simulink model "sf_aircraft"  (Simulink 7.6)
settings: Solver=ode4  StartTime=0.0  StopTime=inf  RelTol=1e-3
PreLoadFcn:
  | noise_factor=1;
  | load sf_aircraft_buses;
undefined symbols (not defined in the file or in its folder): sf_aircraft_ModeType, sigbuilder_block
libraries: simulink x21, sf_aircraft_screen_library x7, simulink_need_slupdate x2
(part 2 of 2)

== system sf_aircraft/Signal conditioning and failures /Actuator Positions/Event Logging/Log LI Actuator  Position Sensors ==
  In1 : Inport
  Enable : EnablePort  PropagateVarSize=During execution
  To Workspace : ToWorkspace  VariableName=LI_log  SampleTime=-1  SaveFormat=Structure With Time
  wires:
  In1/1 -> To Workspace/1  "LI_log"

== system sf_aircraft/Signal conditioning and failures /Actuator Positions/Event Logging/Log LO Actuator  Position Sensors ==
  In1 : Inport
  Enable : EnablePort  PropagateVarSize=During execution
  To Workspace : ToWorkspace  VariableName=LO_log  SampleTime=-1  SaveFormat=Structure With Time
  wires:
  In1/1 -> To Workspace/1  "LO_log"

== system sf_aircraft/Signal conditioning and failures /Actuator Positions/Event Logging/Log RI Actuator  Position Sensors ==
  In1 : Inport
  Enable : EnablePort  PropagateVarSize=During execution
  To Workspace : ToWorkspace  VariableName=RI_log  SampleTime=-1  SaveFormat=Structure With Time
  wires:
  In1/1 -> To Workspace/1  "RO_log"

== system sf_aircraft/Signal conditioning and failures /Actuator Positions/Event Logging/Log RO Actuator  Position Sensors ==
  In1 : Inport
  Enable : EnablePort  PropagateVarSize=During execution
  To Workspace : ToWorkspace  VariableName=RO_log  SampleTime=-1  SaveFormat=Structure With Time
  wires:
  In1/1 -> To Workspace/1  "RI_log"

== system sf_aircraft/Signal conditioning and failures /Hydraulic Pressures/Event Logging/Log Hydraulic System 1 Sensors ==
  In1 : Inport
  Enable : EnablePort  PropagateVarSize=During execution
  To Workspace : ToWorkspace  VariableName=H1_log  SampleTime=-1  SaveFormat=Structure With Time
  wires:
  In1/1 -> To Workspace/1

== system sf_aircraft/Signal conditioning and failures /Hydraulic Pressures/Event Logging/Log Hydraulic System 2 Sensors ==
  In1 : Inport
  Enable : EnablePort  PropagateVarSize=During execution
  To Workspace : ToWorkspace  VariableName=H2_log  SampleTime=-1  SaveFormat=Structure With Time
  wires:
  In1/1 -> To Workspace/1  "H2_log"

== system sf_aircraft/Signal conditioning and failures /Hydraulic Pressures/Event Logging/Log Hydraulic System 3 Sensors ==
  In1 : Inport
  Enable : EnablePort  PropagateVarSize=During execution
  To Workspace : ToWorkspace  VariableName=H3_log  SampleTime=-1  SaveFormat=Structure With Time
  wires:
  In1/1 -> To Workspace/1  "H3_log"

== system sf_aircraft/Signal conditioning and failures /Hydraulic Pressures/Measured  Hydraulic system 1 pressures/Hydraulic pressure ==
  H1_fail : Constant  Value=0  OutDataTypeStr=boolean
  Outlier/failure : Subsystem  Tag=STV Subsys  LoadFcn=sigbuilder_block('load');  StartFcn=sigbuilder_block('start');  StopFcn=sigbuilder_block('stop');  ClipboardFcn=sigbuilder_block('clipboard');  mask(Sigbuilder block){}
      mask help: Sigbuilder GUI
      mask init:
      | if ~strcmp(get_param(bdroot,'SimulationStatus'),'stopped') tuvar = sigbuilder_block('maskInit'); end
      settings: CopyFcn=sigbuilder_block('copy');  DeleteFcn=sigbuilder_block('delete');  ModelCloseFcn=sigbuilder_block('modelClose');  PreSaveFcn=sigbuilder_block('preSave');  NameChangeFcn=sigbuilder_block('namechange');  OpenFcn=sigbuilder_block('open',[81 97.5 519.75 399.75 ]);  CloseFcn=sigbuilder_block('close');
      mask Display: plot(0,0,100,100,[10,10,40,40,10],[80,20,20,80,80],[40,10],[50,50], [40,27,10],[65,72,56],[40,25,25,10],[28,28,43,43]);
  Pump Pressure : Constant  Value=1000
  Switch : Switch  Criteria=u2 ~= 0  SaturateOnIntegerOverflow=on
  Out1 : Outport
  wires:
  Pump Pressure/1 -> Switch/3
  Switch/1 -> Out1/1
  Outlier/failure/1(Signal 1) -> Switch/1
  H1_fail/1 -> Switch/2

== system sf_aircraft/Signal conditioning and failures /Hydraulic Pressures/Measured  Hydraulic system 1 pressures/pressure reading1 ==
  pressure : Inport
  Band-Limited White Noise : simulink/Sources/Band-Limited White Noise  SystemSampleTime=-1  Cov=[0.1]*noise_factor  Ts=0.01  seed=[25341]
  Sum : Sum  Inputs=|++  SaturateOnIntegerOverflow=on
  Out1 : Outport
  wires:
  Sum/1 -> Out1/1
  pressure/1 -> Sum/1
  Band-Limited White Noise/1 -> Sum/2

== system sf_aircraft/Signal conditioning and failures /Hydraulic Pressures/Measured  Hydraulic system 1 pressures/pressure reading2 ==
  pressure : Inport
  Band-Limited White Noise : simulink/Sources/Band-Limited White Noise  SystemSampleTime=-1  Cov=[0.1]*noise_factor  Ts=0.01  seed=[21311]
  Sum1 : Sum  Inputs=|++  SaturateOnIntegerOverflow=on
  Out1 : Outport
  wires:
  Band-Limited White Noise/1 -> Sum1/2
  pressure/1 -> Sum1/1
  Sum1/1 -> Out1/1

== system sf_aircraft/Signal conditioning and failures /Hydraulic Pressures/Measured  Hydraulic system 1 pressures/pressure reading3 ==
  pressure : Inport
  Band-Limited White Noise : simulink/Sources/Band-Limited White Noise  SystemSampleTime=-1  Cov=[0.1]*noise_factor  Ts=0.01  seed=[341]
  Sum1 : Sum  Inputs=|++  SaturateOnIntegerOverflow=on
  Out1 : Outport
  wires:
  Sum1/1 -> Out1/1
  pressure/1 -> Sum1/1
  Band-Limited White Noise/1 -> Sum1/2

== system sf_aircraft/Signal conditioning and failures /Hydraulic Pressures/Measured  Hydraulic system 2 pressures/Hydraulic pressure ==
  H2_fail : Constant  Value=0  OutDataTypeStr=boolean
  Outlier/failure : Subsystem  Tag=STV Subsys  LoadFcn=sigbuilder_block('load');  StartFcn=sigbuilder_block('start');  StopFcn=sigbuilder_block('stop');  ClipboardFcn=sigbuilder_block('clipboard');  mask(Sigbuilder block){}
      mask help: Sigbuilder GUI
      mask init:
      | if ~strcmp(get_param(bdroot,'SimulationStatus'),'stopped') tuvar = sigbuilder_block('maskInit'); end
      settings: CopyFcn=sigbuilder_block('copy');  DeleteFcn=sigbuilder_block('delete');  ModelCloseFcn=sigbuilder_block('modelClose');  PreSaveFcn=sigbuilder_block('preSave');  NameChangeFcn=sigbuilder_block('namechange');  OpenFcn=sigbuilder_block('open',[81 97.5 519.75 399.75 ]);  CloseFcn=sigbuilder_block('close');
      mask Display: plot(0,0,100,100,[10,10,40,40,10],[80,20,20,80,80],[40,10],[50,50], [40,27,10],[65,72,56],[40,25,25,10],[28,28,43,43]);
  Pump Pressure : Constant  Value=1000
  Switch : Switch  Criteria=u2 ~= 0  SaturateOnIntegerOverflow=on
  Out1 : Outport
  wires:
  Pump Pressure/1 -> Switch/3
  Switch/1 -> Out1/1
  Outlier/failure/1(Signal 1) -> Switch/1
  H2_fail/1 -> Switch/2

== system sf_aircraft/Signal conditioning and failures /Hydraulic Pressures/Measured  Hydraulic system 2 pressures/pressure reading1 ==
  pressure : Inport
  Band-Limited White Noise : simulink/Sources/Band-Limited White Noise  SystemSampleTime=-1  Cov=[0.1]*noise_factor  Ts=0.01  seed=[25341]
  Sum : Sum  Inputs=|++  SaturateOnIntegerOverflow=on
  Out1 : Outport
  wires:
  Band-Limited White Noise/1 -> Sum/2
  pressure/1 -> Sum/1
  Sum/1 -> Out1/1

== system sf_aircraft/Signal conditioning and failures /Hydraulic Pressures/Measured  Hydraulic system 2 pressures/pressure reading2 ==
  pressure : Inport
  Band-Limited White Noise : simulink/Sources/Band-Limited White Noise  SystemSampleTime=-1  Cov=[0.1]*noise_factor  Ts=0.01  seed=[21311]
  Sum1 : Sum  Inputs=|++  SaturateOnIntegerOverflow=on
  Out1 : Outport
  wires:
  Sum1/1 -> Out1/1
  pressure/1 -> Sum1/1
  Band-Limited White Noise/1 -> Sum1/2

== system sf_aircraft/Signal conditioning and failures /Hydraulic Pressures/Measured  Hydraulic system 2 pressures/pressure reading3 ==
  pressure : Inport
  Band-Limited White Noise : simulink/Sources/Band-Limited White Noise  SystemSampleTime=-1  Cov=[0.1]*noise_factor  Ts=0.01  seed=[341]
  Sum1 : Sum  Inputs=|++  SaturateOnIntegerOverflow=on
  Out1 : Outport
  wires:
  Band-Limited White Noise/1 -> Sum1/2
  pressure/1 -> Sum1/1
  Sum1/1 -> Out1/1

== system sf_aircraft/Signal conditioning and failures /Hydraulic Pressures/Measured  Hydraulic system 3 pressures/Hydraulic pressure ==
  H3_fail : Constant  Value=0  OutDataTypeStr=boolean
  Outlier/failure : Subsystem  Tag=STV Subsys  LoadFcn=sigbuilder_block('load');  StartFcn=sigbuilder_block('start');  StopFcn=sigbuilder_block('stop');  ClipboardFcn=sigbuilder_block('clipboard');  mask(Sigbuilder block){}
      mask help: Sigbuilder GUI
      mask init:
      | if ~strcmp(get_param(bdroot,'SimulationStatus'),'stopped') tuvar = sigbuilder_block('maskInit'); end
      settings: CopyFcn=sigbuilder_block('copy');  DeleteFcn=sigbuilder_block('delete');  ModelCloseFcn=sigbuilder_block('modelClose');  PreSaveFcn=sigbuilder_block('preSave');  NameChangeFcn=sigbuilder_block('namechange');  OpenFcn=sigbuilder_block('open',[81 97.5 519.75 399.75 ]);  CloseFcn=sigbuilder_block('close');
      mask Display: plot(0,0,100,100,[10,10,40,40,10],[80,20,20,80,80],[40,10],[50,50], [40,27,10],[65,72,56],[40,25,25,10],[28,28,43,43]);
  Pump Pressure : Constant  Value=1000
  Switch : Switch  Criteria=u2 ~= 0  SaturateOnIntegerOverflow=on
  Out1 : Outport
  wires:
  Pump Pressure/1 -> Switch/3
  Switch/1 -> Out1/1
  Outlier/failure/1(Signal 1) -> Switch/1
  H3_fail/1 -> Switch/2

== system sf_aircraft/Signal conditioning and failures /Hydraulic Pressures/Measured  Hydraulic system 3 pressures/pressure reading1 ==
  pressure : Inport
  Band-Limited White Noise : simulink/Sources/Band-Limited White Noise  SystemSampleTime=-1  Cov=[0.1]*noise_factor  Ts=0.01  seed=[2341]
  Sum : Sum  Inputs=|++  SaturateOnIntegerOverflow=on
  Out1 : Outport
  wires:
  Sum/1 -> Out1/1
  pressure/1 -> Sum/1
  Band-Limited White Noise/1 -> Sum/2

== system sf_aircraft/Signal conditioning and failures /Hydraulic Pressures/Measured  Hydraulic system 3 pressures/pressure reading2 ==
  pressure : Inport
  Band-Limited White Noise : simulink/Sources/Band-Limited White Noise  SystemSampleTime=-1  Cov=[0.1]*noise_factor  Ts=0.01  seed=[1311]
  Sum1 : Sum  Inputs=|++  SaturateOnIntegerOverflow=on
  Out1 : Outport
  wires:
  Band-Limited White Noise/1 -> Sum1/2
  pressure/1 -> Sum1/1
  Sum1/1 -> Out1/1

== system sf_aircraft/Signal conditioning and failures /Hydraulic Pressures/Measured  Hydraulic system 3 pressures/pressure reading3 ==
  pressure : Inport
  Band-Limited White Noise : simulink/Sources/Band-Limited White Noise  SystemSampleTime=-1  Cov=[0.1]*noise_factor  Ts=0.01  seed=[1341]
  Sum1 : Sum  Inputs=|++  SaturateOnIntegerOverflow=on
  Out1 : Outport
  wires:
  Sum1/1 -> Out1/1
  pressure/1 -> Sum1/1
  Band-Limited White Noise/1 -> Sum1/2

== system sf_aircraft/Signal conditioning and failures /Hydraulic Pressures/Measured  Hydraulic system 1 pressures/Hydraulic pressure/Outlier/failure ==
  Demux : Demux  Tag=STV Demux  Outputs=1
  FromWs : FromWorkspace  Tag=STV FromWs  VariableName=tuvar  SampleTime=0  SigBuilderData=DataTag8  VnvData=DataTag9
      SigBuilderData=|
      | dataSet.timeRange = [0 30]
      | dataSet.name = 'Group 1'
      | sbobj.Groups.Name = 'Group 1'
      | sbobj.Groups.Signals.Name = 'Signal 1'
      | sbobj.Groups.Signals.XData = [0 30]
      | sbobj.Groups.Signals.YData = [100 100]
      | sbobj.Groups.TimeRange = [0 30]
  Signal 1 : Outport  Tag=STV Outport
  wires:
  FromWs/1 -> Demux/1
  Demux/1 -> Signal 1/1

== system sf_aircraft/Signal conditioning and failures /Hydraulic Pressures/Measured  Hydraulic system 2 pressures/Hydraulic pressure/Outlier/failure ==
  Demux : Demux  Tag=STV Demux  Outputs=1
  FromWs : FromWorkspace  Tag=STV FromWs  VariableName=tuvar  SampleTime=0  SigBuilderData=DataTag10  VnvData=DataTag11
      SigBuilderData=|
      | dataSet.timeRange = [0 30]
      | dataSet.name = 'Group 1'
      | sbobj.Groups.Name = 'Group 1'
      | sbobj.Groups.Signals.Name = 'Signal 1'
      | sbobj.Groups.Signals.XData = [0 30]
      | sbobj.Groups.Signals.YData = [100 100]
      | sbobj.Groups.TimeRange = [0 30]
  Signal 1 : Outport  Tag=STV Outport
  wires:
  FromWs/1 -> Demux/1
  Demux/1 -> Signal 1/1

== system sf_aircraft/Signal conditioning and failures /Hydraulic Pressures/Measured  Hydraulic system 3 pressures/Hydraulic pressure/Outlier/failure ==
  Demux : Demux  Tag=STV Demux  Outputs=1
  FromWs : FromWorkspace  Tag=STV FromWs  VariableName=tuvar  SampleTime=0  SigBuilderData=DataTag12  VnvData=DataTag13
      SigBuilderData=|
      | dataSet.timeRange = [0 30]
      | dataSet.name = 'Group 1'
      | sbobj.Groups.Name = 'Group 1'
      | sbobj.Groups.Signals.Name = 'Signal 1'
      | sbobj.Groups.Signals.XData = [0 30]
      | sbobj.Groups.Signals.YData = [100 100]
      | sbobj.Groups.TimeRange = [0 30]
  Signal 1 : Outport  Tag=STV Outport
  wires:
  FromWs/1 -> Demux/1
  Demux/1 -> Signal 1/1

== stateflow chart Mode Logic ==
  settings: sampleTime=0.5
  state R_switch [function]
    (default) -> (junction 78)
    (junction 78) -> (junction 79) : {
        | /* Hydraulic system 3 Low pressure (Right Outer line) */
        | aVarTruthTableCondition_1 = (u.low_press[2]);
        | }
    (junction 79) -> (junction 80) : {
        | /* Right Outer actuator position failed */
        | aVarTruthTableCondition_2 = (u.R_pos_fail[0]);
        | }
    (junction 80) -> (junction 81) : {
        | /* Hydraulic system 2 Low pressure (Inner line) */
        | aVarTruthTableCondition_3 = (u.low_press[1]);
        | }
    (junction 81) -> (junction 82) : {
        | /* Right Inner actuator position failed */
        | aVarTruthTableCondition_4 = (u.R_pos_fail[1]);
        | }
    (junction 82) -> (junction 83) [order 1] : [aVarTruthTableCondition_1 && !aVarTruthTableCondition_3 && !aVarTruthTableCondition_4]
    (junction 83) -> (junction 84) : {
        | /* Hydraulic System 3 Failure. Turn off Right Outer Actuator */
        | send(go_off,Actuators.RO);
        | }
    (junction 82) -> (junction 85) [order 2]
    (junction 85) -> (junction 86) [order 1] : [aVarTruthTableCondition_1]
    (junction 86) -> (junction 87) : {
        | /* Mulitple Failure. Isolate Right Outer AND Right Inner Actuators */
        | send(go_isolated,Actuators.RO);
        | send(go_isolated,Actuators.RI);
        | }
    (junction 85) -> (junction 88) [order 2]
    (junction 88) -> (junction 89) [order 1] : [!aVarTruthTableCondition_1 && aVarTruthTableCondition_2 && !aVarTruthTableCondition_3 && !aVarTruthTableCondition_4]
    (junction 89) -> (junction 90) : {
        | /* Right Outer Actuator Failure. Isolate Right Outer Actuator */
        | send(go_isolated,Actuators.RO);
        | }
    (junction 88) -> (junction 91) [order 2]
    (junction 91) -> (junction 92) [order 1] : [!aVarTruthTableCondition_1 && aVarTruthTableCondition_2]
    (junction 92) -> (junction 93) : {
        | /* Mulitple Failure. Isolate Right Outer AND Right Inner Actuators */
        | send(go_isolated,Actuators.RO);
        | send(go_isolated,Actuators.RI);
        | }
    (junction 91) -> (junction 94) [order 2]
    (junction 94) -> (junction 95) [order 1] : [aVarTruthTableCondition_3]
    (junction 95) -> (junction 96) : {
        | /* Hydraulic System 2 Failure. Turn off Right Inner Actuator */
        | send(go_off,Actuators.RI);
        | }
    (junction 94) -> (junction 97) [order 2]
    (junction 97) -> (junction 98) [order 1] : [aVarTruthTableCondition_4]
    (junction 98) -> (junction 99) : {
        | /* Right Inner Actuator Failure. Isolate Right Inner Actuator */
        | send(go_isolated,Actuators.RI);
        | }
    (junction 97) -> (junction 100) [order 2]
    (junction 100) -> (junction 101) : /* Default */
    (junction 101) -> (junction 102) : {
        | /* 'Default':Default - All ok, do nothing. */
        |
        | }
  state Actuators
    en:L_switch();R_switch();
    du:L_switch();R_switch();
    state LO [parallel]
      settings: executionOrder=1
      state L1
        state passive
          y.LO_mode=Passive;
        state active
          y.LO_mode=Active;
        state standby
          y.LO_mode=Standby;
        state off
          en:y.LO_mode=Off;
          ex:fails++;
        Actuators.LO.L1.passive -> (junction 45) [order 2]
        Actuators.LO.L1 -> (junction 39) [order 1] : go_off[!in(off)]
        Actuators.LO.L1.off -> Actuators.LO.L1 : [!u.low_press[0]]
        (default) -> Actuators.LO.L1.passive
        Actuators.LO.L1.active -> Actuators.LO.L1.standby : [!RO_act()&&...
            | LI_act()]
        (junction 45) -> Actuators.LO.L1.active : [!LI_act()|RO_act()]
        Actuators.LO.L1.passive -> Actuators.LO.L1.standby [order 1] : [LI_act()]
        Actuators.LO.L1.standby -> (junction 45)
        (junction 39) -> Actuators.LO.L1.off [order 2] : /send(E,LI);
      state isolated
        y.LO_mode=Isolated;
      Actuators.LO.L1 -> Actuators.LO.isolated [order 1] : go_isolated/...
          | send(E,LI);
      (default) -> Actuators.LO.L1
      (junction 39) -> Actuators.LO.isolated [order 1] : [fails>=5]
    state RO [parallel]
      settings: executionOrder=2
      state L1
        state passive
          y.RO_mode=Passive;
        state active
          y.RO_mode=Active;
        state standby
          y.RO_mode=Standby;
        state off
          en:y.RO_mode=Off;
          ex:fails++;
        (junction 52) -> Actuators.RO.L1.active : [!RI_act()|LO_act()]
        Actuators.RO.L1.standby -> (junction 52)
        Actuators.RO.L1.off -> Actuators.RO.L1 : [!u.low_press[2]]
        (junction 51) -> Actuators.RO.L1.off [order 2] : /send(E,RI);
        Actuators.RO.L1 -> (junction 51) [order 1] : go_off[!in(off)]
        Actuators.RO.L1.active -> Actuators.RO.L1.standby : [!LO_act()&&...
            | RI_act()]
        Actuators.RO.L1.passive -> Actuators.RO.L1.standby [order 1] : [RI_act()]
        (default) -> Actuators.RO.L1.passive
        Actuators.RO.L1.passive -> (junction 52) [order 2]
      state isolated
        y.RO_mode=Isolated;
      (default) -> Actuators.RO.L1
      (junction 51) -> Actuators.RO.isolated [order 1] : [fails>=5]
      Actuators.RO.L1 -> Actuators.RO.isolated [order 1] : go_isolated/send(E,RI);
    state LI [parallel]
      settings: executionOrder=3
      state L1
        state passive
          y.LI_mode=Passive;
        state active
          y.LI_mode=Active;
          send(E,LO);
        state standby
          y.LI_mode=Standby;
        state off
          en:y.LI_mode=Off;
          ex:fails++;
        (default) -> Actuators.LI.L1.passive
        Actuators.LI.L1.off -> Actuators.LI.L1 : [!u.low_press[1]]
        (junction 49) -> Actuators.LI.L1.off [order 2] : /send(E,LO);...
            | send(E,RO);
        Actuators.LI.L1 -> (junction 49) [order 1] : go_off[!in(off)]
        Actuators.LI.L1.active -> Actuators.LI.L1.standby : [RO_act()&&...
            | LO_act()]
        Actuators.LI.L1.passive -> Actuators.LI.L1.standby [order 1] : [LO_act()]
        Actuators.LI.L1.standby -> (junction 50)
        (junction 50) -> Actuators.LI.L1.active : [!LO_act()|RI_act()]
        Actuators.LI.L1.passive -> (junction 50) [order 2]
      state isolated
        y.LI_mode=Isolated;
      Actuators.LI.L1 -> Actuators.LI.isolated [order 1] : go_isolated/send(E,LO);...
          | send(E,RO);
      (junction 49) -> Actuators.LI.isolated [order 1] : [fails>=5]
      (default) -> Actuators.LI.L1
    state RI [parallel]
      settings: executionOrder=4
      state L1
        state passive
          y.RI_mode=Passive;
        state active
          y.RI_mode=Active;
          send(E,RO);
        state standby
          y.RI_mode=Standby;
        state off
          en:y.RI_mode=Off;
          ex:fails++;
        Actuators.RI.L1.off -> Actuators.RI.L1 : [!u.low_press[1]]
        (junction 47) -> Actuators.RI.L1.off [order 2] : /send(E,RO);...
            | send(E,LO);send(E,LI);
        Actuators.RI.L1 -> (junction 47) [order 1] : go_off[!in(off)]
        Actuators.RI.L1.active -> Actuators.RI.L1.standby : [LO_act()&&...
            | RO_act()]
        Actuators.RI.L1.passive -> Actuators.RI.L1.standby [order 1] : [RO_act()]
        Actuators.RI.L1.standby -> (junction 48)
        (junction 48) -> Actuators.RI.L1.active : [!RO_act()|LI_act()]
        Actuators.RI.L1.passive -> (junction 48) [order 2]
        (default) -> Actuators.RI.L1.passive
      state isolated
        y.RI_mode=Isolated;
      Actuators.RI.L1 -> Actuators.RI.isolated [order 1] : go_isolated/send(E,RO);...
          | send(E,LO);send(E,LI);
      (junction 47) -> Actuators.RI.isolated [order 1] : [fails>=5]
      (default) -> Actuators.RI.L1
  state y_act = LO_act [function]
    (default) -> (junction 57) : {y_act=in(Actuators.LO.L1.active);}
  state L_switch [function]
    (junction 77) -> (junction 40) : {
        | /* Left Outer actuator position failed */
        | aVarTruthTableCondition_2 = (u.L_pos_fail[0]);
        | }
    (junction 40) -> (junction 41) : {
        | /* Hydraulic system 2 Low pressure (Inner line) */
        | aVarTruthTableCondition_3 = (u.low_press[1]);
        | }
    (junction 41) -> (junction 42) : {
        | /* Left Inner actuator position failed */
        | aVarTruthTableCondition_4 = (u.L_pos_fail[1]);
        | }
    (junction 42) -> (junction 43) [order 1] : [aVarTruthTableCondition_1 && !aVarTruthTableCondition_3 && !aVarTruthTableCondition_4]
    (junction 43) -> (junction 44) : {
        | /* Hydraulic System 1 Failure. Turn off Left Outer Actuator */
        | send(go_off,Actuators.LO);
        | }
    (junction 42) -> (junction 46) [order 2]
    (junction 46) -> (junction 53) [order 1] : [aVarTruthTableCondition_1]
    (junction 53) -> (junction 54) : {
        | /* Left Outer Actuator Failure. Isolate Left Outer Actuator */
        | send(go_isolated,Actuators.LO);
        | }
    (junction 54) -> (junction 59) : {
        | /* Left Inner Actuator Failure. Isolate Left Inner Actuator */
        | send(go_isolated,Actuators.LI);
        | }
    (junction 46) -> (junction 60) [order 2]
    (junction 60) -> (junction 61) [order 1] : [!aVarTruthTableCondition_1 && aVarTruthTableCondition_2 && !aVarTruthTableCondition_3 && !aVarTruthTableCondition_4]
    (junction 61) -> (junction 62) : {
        | /* Left Outer Actuator Failure. Isolate Left Outer Actuator */
        | send(go_isolated,Actuators.LO);
        | }
    (junction 60) -> (junction 63) [order 2]
    (junction 63) -> (junction 64) [order 1] : [!aVarTruthTableCondition_1 && aVarTruthTableCondition_2]
    (junction 64) -> (junction 65) : {
        | /* Left Outer Actuator Failure. Isolate Left Outer Actuator */
        | send(go_isolated,Actuators.LO);
        | }
    (junction 65) -> (junction 66) : {
        | /* Left Inner Actuator Failure. Isolate Left Inner Actuator */
        | send(go_isolated,Actuators.LI);
        | }
    (junction 63) -> (junction 67) [order 2]
    (junction 67) -> (junction 68) [order 1] : [aVarTruthTableCondition_3]
    (junction 68) -> (junction 69) : {
        | /* Hydraulic System 2 Failure. Turn off Left Inner Actuator */
        | send(go_off,Actuators.LI);
        | }
    (junction 67) -> (junction 70) [order 2]
    (junction 70) -> (junction 71) [order 1] : [aVarTruthTableCondition_4]
    (junction 71) -> (junction 72) : {
        | /* Left Inner Actuator Failure. Isolate Left Inner Actuator */
        | send(go_isolated,Actuators.LI);
        | }
    (junction 70) -> (junction 73) [order 2]
    (junction 73) -> (junction 74) : /* Default */
    (junction 74) -> (junction 75) : {
        | /* 'Default':Default - All ok, do nothing. */
        |
        | }
    (default) -> (junction 76)
    (junction 76) -> (junction 77) : {
        | /* Hydraulic system 1 Low pressure (Left Outer line) */
        | aVarTruthTableCondition_1 = (u.low_press[0]);
        | }
  note: This mode logic assumes that there are 3 hydraulic lines, one that is connected to the 2 redundant actuators (Left Inner and Right Inner actuators).
      | The other two are connected to the primary actuators Left Outer and Right Outer (1 per actuator).
  state y_act = RI_act [function]
    (default) -> (junction 55) : {y_act=in(Actuators.RI.L1.active);}
  state y_act = RO_act [function]
    (default) -> (junction 56) : {y_act=in(Actuators.RO.L1.active);}
  state y_act = LI_act [function]
    (default) -> (junction 58) : {y_act=in(Actuators.LI.L1.active);}
  data: aVarTruthTableCondition_1 temporary boolean =0; aVarTruthTableCondition_2 temporary boolean =0; aVarTruthTableCondition_3 temporary boolean =0; aVarTruthTableCondition_4 temporary boolean =0; y_act function_output double; fails local int32; aVarTruthTableCondition_1 temporary boolean =0; aVarTruthTableCondition_2 temporary boolean =0; aVarTruthTableCondition_3 temporary boolean =0; aVarTruthTableCondition_4 temporary boolean =0; y_act function_output double; y_act function_output double; y_act function_output double; fails local int32; fails local int32; fails local int32; u input Bus: PositionBus size=1; y output ModeBus
  data aVarTruthTableCondition_1 settings: description=Hydraulic system 3 Low pressure (Right Outer line)
  data aVarTruthTableCondition_2 settings: description=Right Outer actuator position failed
  data aVarTruthTableCondition_3 settings: description=Hydraulic system 2 Low pressure (Inner line)
  data aVarTruthTableCondition_4 settings: description=Right Inner actuator position failed
  data aVarTruthTableCondition_1 settings: description=Hydraulic system 1 Low pressure (Left Outer line)
  data aVarTruthTableCondition_2 settings: description=Left Outer actuator position failed
  data aVarTruthTableCondition_3 settings: description=Hydraulic system 2 Low pressure (Inner line)
  data aVarTruthTableCondition_4 settings: description=Left Inner actuator position failed
  events: go_isolated local EITHER_EDGE_EVENT; go_off local EITHER_EDGE_EVENT; E local EITHER_EDGE_EVENT
